simulink model "VibrationAbsorber"  (R2020b)
settings: Solver=VariableStepAuto  StartTime=0.0  StopTime=10.0  RelTol=1e-3
model workspace (MAT data in the model file):
  M1 = 100
  M2 = 100
  b = 50
  k1 = 50
  k12 = 10000
settings Model: Creator=abhin  LastModifiedBy=abhin

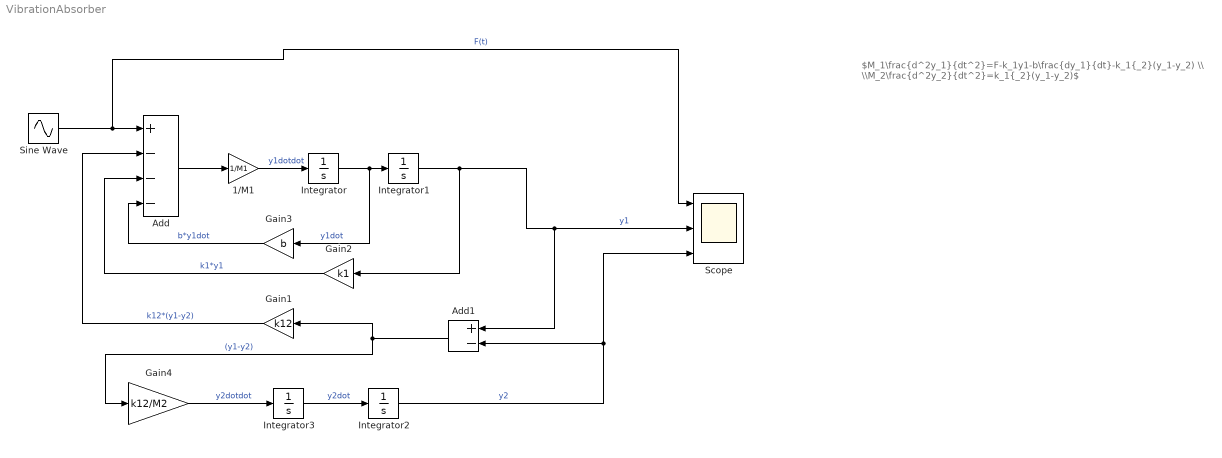
== system VibrationAbsorber ==
  note: $M_1\frac{d^2y_1}{dt^2}=F-k_1y1-b\frac{dy_1}{dt}-k_1{_2}(y_1-y_2) \\ \\M_2\frac{d^2y_2}{dt^2}=k_1{_2}(y_1-y_2)$
  1/M1 : Gain  Gain=1/M1
  Add : Sum  Inputs=+---
  Add1 : Sum  Inputs=+-
  Gain1 : Gain  Gain=k12
  Gain2 : Gain  Gain=k1
  Gain3 : Gain  Gain=b
  Gain4 : Gain  Gain=k12/M2
  Integrator{,1..3} (4 alike) : Integrator
  Scope : Scope  NumInputPorts=3
  Sine Wave : Sin  Amplitude=2  Frequency=10  SampleTime=0.001
  wires:
  Gain1/1 -> Add/2  "k12*(y1-y2)"
  Add1/1 -> Gain4/1, Gain1/1  "(y1-y2)"
  Gain4/1 -> Integrator3/1  "y2dotdot"
  1/M1/1 -> Integrator/1  "y1dotdot"
  Gain2/1 -> Add/3  "k1*y1"
  Gain3/1 -> Add/4  "b*y1dot"
  Integrator3/1 -> Integrator2/1  "y2dot"
  Sine Wave/1 -> Scope/1, Add/1  "F(t)"
  Integrator2/1 -> Add1/2, Scope/3  "y2"
  Integrator/1 -> Gain3/1, Integrator1/1  "y1dot"
  Integrator1/1 -> Gain2/1, Scope/2, Add1/1  "y1"
  Add/1 -> 1/M1/1
